simulink model "assignment4"  (R2016a)
settings: Solver=VariableStepAuto  StartTime=0.0  StopTime=10.0  RelTol=1e-3
libraries: simulink_extras x4
settings Model: Creator=Sondre  LastModifiedBy=Sondre

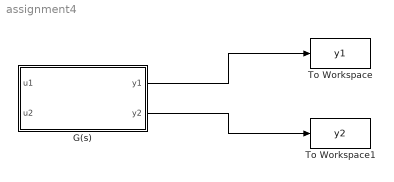
== system assignment4 ==
  G(s) : Subsystem
  To Workspace : ToWorkspace  VariableName=y1  SaveFormat=Timeseries  SampleTime=-1
  To Workspace1 : ToWorkspace  VariableName=y2  SaveFormat=Timeseries  SampleTime=-1
  wires:
  G(s)/1(y1) -> To Workspace/1
  G(s)/2(y2) -> To Workspace1/1

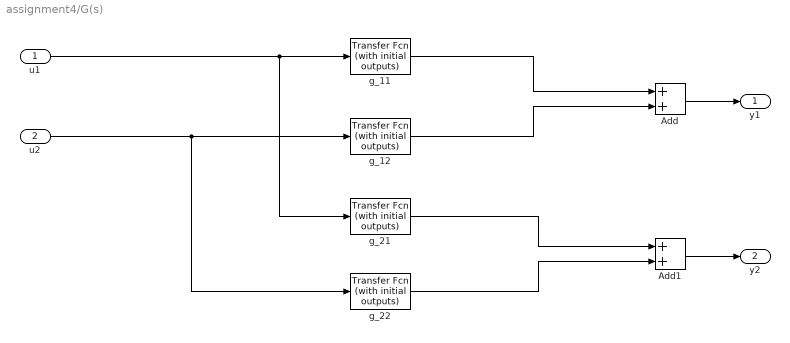
== system assignment4/G(s) ==
  u1 : Inport
  u2 : Inport  Port=2
  Add : Sum
  Add1 : Sum
  g_11 : simulink_extras/Additional Linear/Transfer Fcn (with initial outputs)  N=[3 6]  D="[1  4 3]"  Y0=.5  U0=0
  g_12 : simulink_extras/Additional Linear/Transfer Fcn (with initial outputs)  N=[2]  D=[1 1]  Y0=.5  U0=0
  g_21 : simulink_extras/Additional Linear/Transfer Fcn (with initial outputs)  N=[1]  D=[1 2]  Y0=.5  U0=0
  "g_22 " : simulink_extras/Additional Linear/Transfer Fcn (with initial outputs)  N=[1]  D=[1 3]  Y0=.5  U0=0
  y1 : Outport
  y2 : Outport  Port=2
  wires:
  Add/1 -> y1/1
  g_11/1 -> Add/1
  g_12/1 -> Add/2
  u2/1 -> "g_22 "/1, g_12/1
  Add1/1 -> y2/1
  u1/1 -> g_21/1, g_11/1
  g_21/1 -> Add1/1
  "g_22 "/1 -> Add1/2
